simulink model "zrf_test"  (R2019a)
settings: Solver=VariableStepAuto  StartTime=0.0  StopTime=10.0  RelTol=1e-3
libraries: xbsIndex_r4 x3314, casper_library_misc x18, xps_library x3
(part 1 of 32)
settings Model: Creator=jackh  LastModifiedBy=jackh

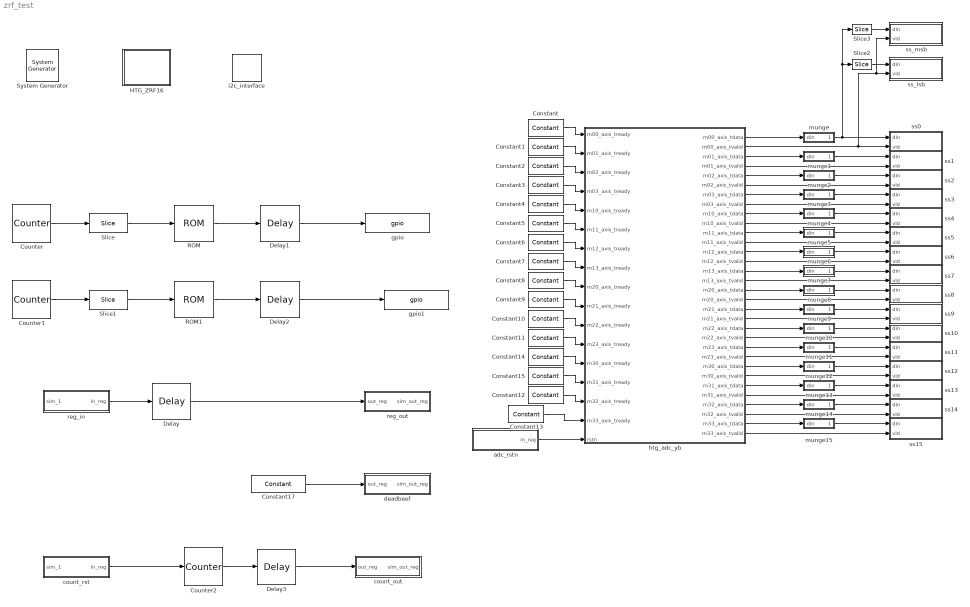
== system zrf_test ==
  " System Generator" : xbsIndex_r4/ System Generator  Tag=genX  xilinxfamily=zynquplusRFSOC  part=xczu49dr  speed=-2-e  package=ffvf1760  synthesis_tool=XST  clock_wrapper=Clock Enables  directory=/home/jackh/src/ata_rfsoc/zrf_test/sysgen  proj_type=Vivado  Synth_file=Vivado Synthesis Defaults  Impl_file=Vivado Implementation Defaults  testbench=off  simulink_period=1  sysclk_period=3.9062  dcm_input_clock_period=10  incr_netlist=off  trim_vbits=Everywhere in SubSystem  dbl_ovrd=According to Block Masks  core_generation=According to Block Masks  run_coregen=off  deprecated_control=off  eval_field=0  block_type=sysgen
  Constant{,1..15} (16 alike) : xbsIndex_r4/Constant  const=1  gui_display_data_type=Boolean  arith_type=Boolean  n_bits=1  bin_pt=0  preci_type=Single  exp_width=8  frac_width=24  explicit_period=on  period=1  equ=P=C  opselect=C  inp2=PCIN>>17  opr=+  inp1=P  carry=CIN  dbl_ovrd=off  block_type=constant
  Constant17 : xbsIndex_r4/Constant  const=hex2dec('deadbeef')  gui_display_data_type=Fixed-point  arith_type=Unsigned  n_bits=32  bin_pt=0  preci_type=Single  exp_width=8  frac_width=24  explicit_period=on  period=1  equ=P=C  opselect=C  inp2=PCIN>>17  opr=+  inp1=P  carry=CIN  dbl_ovrd=off  block_type=constant
  Counter : xbsIndex_r4/Counter  cnt_type=Free Running  cnt_to=Inf  operation=Up  start_count=0  cnt_by_val=1  arith_type=Unsigned  n_bits=32  bin_pt=0  load_pin=off  rst=off  en=off  explicit_period=on  period=1  use_behavioral_HDL=off  implementation=Fabric  dbl_ovrd=off  block_type=counter
  Counter1 : xbsIndex_r4/Counter  cnt_type=Free Running  cnt_to=Inf  operation=Up  start_count=0  cnt_by_val=1  arith_type=Unsigned  n_bits=32  bin_pt=0  load_pin=off  rst=off  en=off  explicit_period=on  period=1  use_behavioral_HDL=off  implementation=Fabric  dbl_ovrd=off  block_type=counter
  Counter2 : xbsIndex_r4/Counter  cnt_type=Free Running  cnt_to=Inf  operation=Up  start_count=0  cnt_by_val=1  arith_type=Unsigned  n_bits=32  bin_pt=0  load_pin=off  rst=on  en=off  explicit_period=on  period=1  use_behavioral_HDL=off  implementation=DSP48  dbl_ovrd=off  block_type=counter
  Delay{,1..3} (4 alike) : xbsIndex_r4/Delay  rst=off  infoeditControl=Selection of Reset will increase slice count due to use of real FFs and instead of SRLs  en=off  latency=1  reg_retiming=off  dbl_ovrd=off  block_type=delay
  HTG_ZRF16 : Subsystem  Tag=xps:xsg  mask(xsg core config){hw_sys=htg_zrf16:xczu49dr, clk_src=adc_clk, clk_rate=256, sample_period=1, synthesis_tool=XST}
      mask prompts: hw_sys "Hardware Platform"; clk_src "User IP Clock source"; clk_rate "User IP Clock Rate (MHz)"; sample_period "Sample Period"; synthesis_tool "Synthesis Tool:"
      mask help:
      | The XSG Core Config block is used to configure the System Generator design
      | for the casper_xps toolflow. Settings here are used to configure the
      | Xilinx System Generator block parameters automatically, and control toolflow
      | script  execution. It needs to be at the top level of all designs being compiled
      | with the casper_xps toolflow.
      mask init:
      | xps_xsg_htg_zrf16_conf_mask;
      mask Help: eval('xlWeb([getenv(''MLIB_ROOT''), ''\doc\html\sys_xsg_core_config\sys_xsg_core_config.html''])')
      mask TypeOptions hw_sys: htg_zrf16:xczu29dr | htg_zrf16:xczu49dr
      mask TypeOptions clk_src: sys_clk | adc_clk | arb_clk
      mask TypeOptions synthesis_tool: Leonardo Spectrum | Synplify | Synplify Pro | XST
      mask Display: fprintf(['ZRF16']);
  ROM : xbsIndex_r4/ROM  depth=16  initVector=[0 1 2 4 8 16 32 64 64 32 16 8 4 2 1 0]  distributed_mem=Distributed memory  rst=off  init_reg=0  en=off  latency=1  gui_display_data_type=Fixed-point  arith_type=Unsigned  n_bits=7  bin_pt=0  preci_type=Single  exp_width=8  frac_width=24  optimize=Area  use_rpm=on  dbl_ovrd=off  simulation_type=fast_sim  block_type=sprom
  ROM1 : xbsIndex_r4/ROM  depth=16  initVector=[1 2 4 8 16 32 64 128 128 64 32 16 8 4 2 1]  distributed_mem=Distributed memory  rst=off  init_reg=0  en=off  latency=1  gui_display_data_type=Fixed-point  arith_type=Unsigned  n_bits=8  bin_pt=0  preci_type=Single  exp_width=8  frac_width=24  optimize=Area  use_rpm=on  dbl_ovrd=off  simulation_type=fast_sim  block_type=sprom
  Slice : xbsIndex_r4/Slice  nbits=4  boolean_output=off  mode=Lower Bit Location + Width  bit1=0  base1=MSB of Input  bit0=25  base0=LSB of Input  dbl_ovrd=off  block_type=slice
  Slice1 : xbsIndex_r4/Slice  nbits=4  boolean_output=off  mode=Lower Bit Location + Width  bit1=0  base1=MSB of Input  bit0=25  base0=LSB of Input  dbl_ovrd=off  block_type=slice
  Slice2 : xbsIndex_r4/Slice  nbits=8  boolean_output=off  mode=Lower Bit Location + Width  bit1=0  base1=MSB of Input  bit0=0  base0=LSB of Input  dbl_ovrd=off  block_type=slice
  Slice3 : xbsIndex_r4/Slice  nbits=8  boolean_output=off  mode=Lower Bit Location + Width  bit1=0  base1=MSB of Input  bit0=8  base0=LSB of Input  dbl_ovrd=off  block_type=slice
  adc_rstn : Subsystem  Tag=xps:sw_reg  AncestorBlock=xps_library/Memory/software_register  mask(swreg){io_dir=From Processor, io_delay=0, init_val=0, sample_period=1, names=reg, bitwidths=1, bin_pts=0, arith_types=2, sim_port=off, show_format=on}
      mask prompts: io_dir "I/O direction"; io_delay "I/O delay"; init_val "Initial Value"; sample_period "Sample period"; names "Bitfield names [msb...lsb]"; bitwidths "Bitfield widths"; bin_pts "Bitfield binary pts"; arith_types "Bitfield types, ufix=0, fix=1, bool=2"; sim_port "Provide sim input/output?"; show_format "Print format string?"
      mask help: A 32-bit software-accessible register. Can be divided into bitfields of varying widths and types using the fields in the block mask.
      mask init:
      | swreg_init(gcb)
      settings: AttributesFormatString=1input:b = 1 bits
      mask TypeOptions io_dir: To Processor | From Processor
      mask Callback io_dir:
      | mask_enables = get_param(gcb, 'MaskEnables');
      | mask_names = get_param(gcb, 'MaskNames');
      | if strcmp(get_param(gcb, 'io_dir'), 'To Processor'),
      |     mask_enables{ismember(mask_names, 'sample_period')} = 'off';
      | else
      |     mask_enables{ismember(mask_names, 'sample_period')} = 'on';
      | end
      | set_param(gcb, 'MaskEnables', mask_enables);
      mask DialogControl ParameterTabVar0 Prompt: Setup
  count_out : Subsystem  Tag=xps:sw_reg  AncestorBlock=xps_library/Memory/software_register  mask(swreg){io_dir=To Processor, io_delay=0, init_val=0, sample_period=1, names=reg, bitwidths=32, bin_pts=0, arith_types=0, sim_port=on, show_format=on}
      mask prompts: io_dir "I/O direction"; io_delay "I/O delay"; init_val "Initial Value"; sample_period "Sample period"; names "Bitfield names [msb...lsb]"; bitwidths "Bitfield widths"; bin_pts "Bitfield binary pts"; arith_types "Bitfield types, ufix=0, fix=1, bool=2"; sim_port "Provide sim input/output?"; show_format "Print format string?"
      mask help: A 32-bit software-accessible register. Can be divided into bitfields of varying widths and types using the fields in the block mask.
      mask init:
      | swreg_init(gcb)
      settings: AttributesFormatString=1output:uf32.0 = 32 bits
      mask TypeOptions io_dir: To Processor | From Processor
      mask Callback io_dir:
      | mask_enables = get_param(gcb, 'MaskEnables');
      | mask_names = get_param(gcb, 'MaskNames');
      | if strcmp(get_param(gcb, 'io_dir'), 'To Processor'),
      |     mask_enables{ismember(mask_names, 'sample_period')} = 'off';
      | else
      |     mask_enables{ismember(mask_names, 'sample_period')} = 'on';
      | end
      | set_param(gcb, 'MaskEnables', mask_enables);
      mask DialogControl ParameterTabVar0 Prompt: Setup
  count_rst : Subsystem  Tag=xps:sw_reg  AncestorBlock=xps_library/Memory/software_register  mask(swreg){io_dir=From Processor, io_delay=0, init_val=0, sample_period=1, names=reg, bitwidths=1, bin_pts=0, arith_types=2, sim_port=on, show_format=on}
      mask prompts: io_dir "I/O direction"; io_delay "I/O delay"; init_val "Initial Value"; sample_period "Sample period"; names "Bitfield names [msb...lsb]"; bitwidths "Bitfield widths"; bin_pts "Bitfield binary pts"; arith_types "Bitfield types, ufix=0, fix=1, bool=2"; sim_port "Provide sim input/output?"; show_format "Print format string?"
      mask help: A 32-bit software-accessible register. Can be divided into bitfields of varying widths and types using the fields in the block mask.
      mask init:
      | swreg_init(gcb)
      settings: AttributesFormatString=1input:b = 1 bits
      mask TypeOptions io_dir: To Processor | From Processor
      mask Callback io_dir:
      | mask_enables = get_param(gcb, 'MaskEnables');
      | mask_names = get_param(gcb, 'MaskNames');
      | if strcmp(get_param(gcb, 'io_dir'), 'To Processor'),
      |     mask_enables{ismember(mask_names, 'sample_period')} = 'off';
      | else
      |     mask_enables{ismember(mask_names, 'sample_period')} = 'on';
      | end
      | set_param(gcb, 'MaskEnables', mask_enables);
      mask DialogControl ParameterTabVar0 Prompt: Setup
  deadbeef : Subsystem  Tag=xps:sw_reg  AncestorBlock=xps_library/Memory/software_register  mask(swreg){io_dir=To Processor, io_delay=0, init_val=0, sample_period=1, names=reg, bitwidths=32, bin_pts=0, arith_types=0, sim_port=on, show_format=on}
      mask prompts: io_dir "I/O direction"; io_delay "I/O delay"; init_val "Initial Value"; sample_period "Sample period"; names "Bitfield names [msb...lsb]"; bitwidths "Bitfield widths"; bin_pts "Bitfield binary pts"; arith_types "Bitfield types, ufix=0, fix=1, bool=2"; sim_port "Provide sim input/output?"; show_format "Print format string?"
      mask help: A 32-bit software-accessible register. Can be divided into bitfields of varying widths and types using the fields in the block mask.
      mask init:
      | swreg_init(gcb)
      settings: AttributesFormatString=1output:uf32.0 = 32 bits
      mask TypeOptions io_dir: To Processor | From Processor
      mask Callback io_dir:
      | mask_enables = get_param(gcb, 'MaskEnables');
      | mask_names = get_param(gcb, 'MaskNames');
      | if strcmp(get_param(gcb, 'io_dir'), 'To Processor'),
      |     mask_enables{ismember(mask_names, 'sample_period')} = 'off';
      | else
      |     mask_enables{ismember(mask_names, 'sample_period')} = 'on';
      | end
      | set_param(gcb, 'MaskEnables', mask_enables);
      mask DialogControl ParameterTabVar0 Prompt: Setup
  gpio : xps_library/IO/gpio  Tag=xps:gpio  io_group_params_forwarded=off  io_group=ROACH:led  io_group_real=led  io_group_custom=0  io_dir=out  arith_type=Unsigned  bitwidth=7  bin_pt=0  bit_index=[0 1 2 3 4 5 6]  sample_period=1  use_single_ended=off  use_ddr=off  reg_iob=on  reg_clk_phase=0  termination=None
      settings: SourceProductName=CASPER XPS Blockset
  gpio1 : xps_library/IO/gpio  Tag=xps:gpio  io_group_params_forwarded=off  io_group=ROACH:led  io_group_real=gpio  io_group_custom=0  io_dir=out  arith_type=Unsigned  bitwidth=8  bin_pt=0  bit_index=[0 1 2 3 4 5 6 7]  sample_period=1  use_single_ended=off  use_ddr=off  reg_iob=on  reg_clk_phase=0  termination=None
      settings: SourceProductName=CASPER XPS Blockset
  htg_adc_yb : Subsystem  Tag=xps:adc_htgzrf16  mask(htg_adc){tile_224_enable_pll=on, tile_224_sample_rate=4096, tile_224_clk_out=256.000, tile_224_ref_clk=512.000, tile_224_axi_stream_clk=0, tile_224_adc_0=on, tile_224_adc0_digital_output=I/Q, tile_224_adc0_dec_mode=2x, tile_224_adc0_sample_per_cycle=8, tile_224_adc0_req_axis_clk=0, tile_224_adc_1=on, tile_224_adc1_digital_output=I/Q, tile_224_adc1_dec_mode=2x, tile_224_adc1_sample_per_cycle=8, tile_224_adc1_req_axis_clk=0, tile_225_enable_pll=on, tile_225_sample_rate=4096, tile_225_clk_out=256.000, tile_225_ref_clk=512.000, tile_225_axi_stream_clk=0, tile_225_adc_0=on, tile_225_adc0_digital_output=I/Q, tile_225_adc0_dec_mode=2x, tile_225_adc0_sample_per_cycle=8, tile_225_adc0_req_axis_clk=0, tile_225_adc_1=on, tile_225_adc1_digital_output=I/Q, tile_225_adc1_dec_mode=2x, tile_225_adc1_sample_per_cycle=8, tile_225_adc1_req_axis_clk=0, tile_226_enable_pll=on, tile_226_sample_rate=4096, tile_226_clk_out=256.000, tile_226_ref_clk=512.000, tile_226_axi_stream_clk=0, tile_226_adc_0=on, tile_226_adc0_digital_output=I/Q, tile_226_adc0_dec_mode=2x, tile_226_adc0_sample_per_cycle=8, tile_226_adc0_req_axis_clk=0, tile_226_adc_1=on, tile_226_adc1_digital_output=I/Q, tile_226_adc1_dec_mode=2x, tile_226_adc1_sample_per_cycle=8, tile_226_adc1_req_axis_clk=0, tile_227_enable_pll=on, tile_227_sample_rate=4096, tile_227_clk_out=256.000, tile_227_ref_clk=512.000, tile_227_axi_stream_clk=0, tile_227_adc_0=on, tile_227_adc0_digital_output=I/Q, tile_227_adc0_dec_mode=2x, tile_227_adc0_sample_per_cycle=8, tile_227_adc0_req_axis_clk=0, tile_227_adc_1=on, tile_227_adc1_digital_output=I/Q, tile_227_adc1_dec_mode=2x, tile_227_adc1_sample_per_cycle=8, tile_227_adc1_req_axis_clk=0}
      mask prompts: tile_224_enable_pll "Enable PLL"; tile_224_sample_rate "Sampling Rate (MSPS)"; tile_224_clk_out "Clock Out (MHz)"; tile_224_ref_clk "Reference Clock (MHz)"; tile_224_axi_stream_clk "AXI4-Stream Clock (MHz)"; tile_224_adc_0 "Enable ADC"; tile_224_adc0_digital_output "Digital Output Data"; tile_224_adc0_dec_mode "Decimation Mode"; tile_224_adc0_sample_per_cycle "Samples per AXI4-Stream Cycle"; tile_224_adc_1 "Enable ADC"; tile_224_adc1_digital_output "Digital Output Data"; tile_224_adc1_dec_mode "Decimation Mode"; tile_224_adc1_sample_per_cycle "Samples per AXI4-Stream Cycle"; tile_225_enable_pll "Enable PLL"; tile_225_sample_rate "Sampling Rate (MSPS)"; tile_225_clk_out "Clock Out (MHz)"; tile_225_ref_clk "Reference Clock (MHz)"; tile_225_axi_stream_clk "AXI4-Stream Clock (MHz)"; tile_225_adc_0 "Enable ADC"; tile_225_adc0_digital_output "Digital Output Data"; tile_225_adc0_dec_mode "Decimation Mode"; tile_225_adc0_sample_per_cycle "Samples per AXI4-Stream Cycle"; tile_225_adc_1 "Enable ADC"; tile_225_adc1_digital_output "Digital Output Data"; tile_225_adc1_dec_mode "Decimation Mode"; tile_225_adc1_sample_per_cycle "Samples per AXI4-Stream Cycle"; tile_226_enable_pll "Enable PLL"; tile_226_sample_rate "Sampling Rate (MSPS)"; tile_226_clk_out "Clock Out (MHz)"; tile_226_ref_clk "Reference Clock (MHz)"; tile_226_axi_stream_clk "AXI4-Stream Clock (MHz)"; tile_226_adc_0 "Enable ADC"; tile_226_adc0_digital_output "Digital Output Data"; tile_226_adc0_dec_mode "Decimation Mode"; tile_226_adc0_sample_per_cycle "Samples per AXI4-Stream Cycle"; tile_226_adc_1 "Enable ADC"; tile_226_adc1_digital_output "Digital Output Data"; tile_226_adc1_dec_mode "Decimation Mode"; tile_226_adc1_sample_per_cycle "Samples per AXI4-Stream Cycle"; tile_227_enable_pll "Enable PLL"; tile_227_sample_rate "Sampling Rate (MSPS)"; tile_227_clk_out "Clock Out (MHz)"; tile_227_ref_clk "Reference Clock (MHz)"; tile_227_axi_stream_clk "AXI4-Stream Clock (MHz)"; tile_227_adc_0 "Enable ADC"; tile_227_adc0_digital_output "Digital Output Data"; tile_227_adc0_dec_mode "Decimation Mode"; tile_227_adc0_sample_per_cycle "Samples per AXI4-Stream Cycle"; tile_227_adc_1 "Enable ADC"; tile_227_adc1_digital_output "Digital Output Data"; tile_227_adc1_dec_mode "Decimation Mode"; tile_227_adc1_sample_per_cycle "Samples per AXI4-Stream Cycle"
      mask init:
      | htg_adc_mask(gcb)
      mask Help: eval('xlWeb([getenv(''MLIB_ROOT''), ''\doc\html\adc_zcu111\adc_zcu111.html''])')
      mask TypeOptions tile_224_clk_out: 32.000 | 64.000 | 128.000 | 256.000
      mask TypeOptions tile_224_ref_clk: 103.261 | 104.136 | 105.026 | 105.931 | 106.852 | 107.790 | 108.743 | 109.714 | 110.703 | 111.709 | 112.734 | 113.778 | 114.841 | 115.925 | 117.029 | 118.154 | 119.301 | 120.471 | 121.663 | 122.880 | 124.121 | 125.388 | 126.680 | 128.000 | 129.347 | 130.723 | 132.129 | 133.565 | 135.033 | 136.533 | 138.067 | 139.636 | 141.241 | 142.884 | 144.565 | 146.286 | 148.048 | 149.854 | 151.704 | 153.600 | 155.544 | 157.539 | 159.584 | 161.684 | 163.840 | 166.054 | 168.329 | 170.667 | 173.070 | 175.543 | 178.087 | 180.706 | 183.403 | 186.182 | 189.046 | 192.000 | 195.048 | 198.194 | 201.443 | 204.800 | 208.271 | 211.862 | 215.579 | 219.429 | 223.418 | 227.556 | 231.849 | 236.308 | 240.941 | 245.760 | 250.776 | 256.000 | 261.447 | 267.130 | 273.067 | 279.273 | 285.767 | 292.571 | 299.707 | 307.200 | 315.077 | 323.368 | 332.108 | 341.333 | 351.086 | 361.412 | 372.364 | 384.000 | 396.387 | 409.600 | 423.724 | 438.857 | 455.111 | 472.615 | 491.520 | 512.000 | 534.261 | 558.546 | 585.143 | 614.400 | 646.737 | 682.667 | 722.824 | 768.000
      mask TypeOptions tile_224_adc0_digital_output: I/Q | Real
      mask TypeOptions tile_224_adc0_dec_mode: 1x | 2x | 4x | 8x
      mask TypeOptions tile_224_adc0_sample_per_cycle: 1 | 2 | 3 | 4 | 5 | 6 | 7 | 8
      mask TypeOptions tile_224_adc1_digital_output: I/Q | Real
      mask TypeOptions tile_224_adc1_dec_mode: 1x | 2x | 4x | 8x
      mask TypeOptions tile_224_adc1_sample_per_cycle: 1 | 2 | 3 | 4 | 5 | 6 | 7 | 8
      mask TypeOptions tile_225_clk_out: 32.000 | 64.000 | 128.000 | 256.000
      mask TypeOptions tile_225_ref_clk: 103.261 | 104.136 | 105.026 | 105.931 | 106.852 | 107.790 | 108.743 | 109.714 | 110.703 | 111.709 | 112.734 | 113.778 | 114.841 | 115.925 | 117.029 | 118.154 | 119.301 | 120.471 | 121.663 | 122.880 | 124.121 | 125.388 | 126.680 | 128.000 | 129.347 | 130.723 | 132.129 | 133.565 | 135.033 | 136.533 | 138.067 | 139.636 | 141.241 | 142.884 | 144.565 | 146.286 | 148.048 | 149.854 | 151.704 | 153.600 | 155.544 | 157.539 | 159.584 | 161.684 | 163.840 | 166.054 | 168.329 | 170.667 | 173.070 | 175.543 | 178.087 | 180.706 | 183.403 | 186.182 | 189.046 | 192.000 | 195.048 | 198.194 | 201.443 | 204.800 | 208.271 | 211.862 | 215.579 | 219.429 | 223.418 | 227.556 | 231.849 | 236.308 | 240.941 | 245.760 | 250.776 | 256.000 | 261.447 | 267.130 | 273.067 | 279.273 | 285.767 | 292.571 | 299.707 | 307.200 | 315.077 | 323.368 | 332.108 | 341.333 | 351.086 | 361.412 | 372.364 | 384.000 | 396.387 | 409.600 | 423.724 | 438.857 | 455.111 | 472.615 | 491.520 | 512.000 | 534.261 | 558.546 | 585.143 | 614.400 | 646.737 | 682.667 | 722.824 | 768.000
      mask TypeOptions tile_225_adc0_digital_output: I/Q | Real
      mask TypeOptions tile_225_adc0_dec_mode: 1x | 2x | 4x | 8x
      mask TypeOptions tile_225_adc0_sample_per_cycle: 1 | 2 | 3 | 4 | 5 | 6 | 7 | 8
      mask TypeOptions tile_225_adc1_digital_output: I/Q | Real
      mask TypeOptions tile_225_adc1_dec_mode: 1x | 2x | 4x | 8x
      mask TypeOptions tile_225_adc1_sample_per_cycle: 1 | 2 | 3 | 4 | 5 | 6 | 7 | 8
      mask TypeOptions tile_226_clk_out: 32.000 | 64.000 | 128.000 | 256.000
      mask TypeOptions tile_226_ref_clk: 103.261 | 104.136 | 105.026 | 105.931 | 106.852 | 107.790 | 108.743 | 109.714 | 110.703 | 111.709 | 112.734 | 113.778 | 114.841 | 115.925 | 117.029 | 118.154 | 119.301 | 120.471 | 121.663 | 122.880 | 124.121 | 125.388 | 126.680 | 128.000 | 129.347 | 130.723 | 132.129 | 133.565 | 135.033 | 136.533 | 138.067 | 139.636 | 141.241 | 142.884 | 144.565 | 146.286 | 148.048 | 149.854 | 151.704 | 153.600 | 155.544 | 157.539 | 159.584 | 161.684 | 163.840 | 166.054 | 168.329 | 170.667 | 173.070 | 175.543 | 178.087 | 180.706 | 183.403 | 186.182 | 189.046 | 192.000 | 195.048 | 198.194 | 201.443 | 204.800 | 208.271 | 211.862 | 215.579 | 219.429 | 223.418 | 227.556 | 231.849 | 236.308 | 240.941 | 245.760 | 250.776 | 256.000 | 261.447 | 267.130 | 273.067 | 279.273 | 285.767 | 292.571 | 299.707 | 307.200 | 315.077 | 323.368 | 332.108 | 341.333 | 351.086 | 361.412 | 372.364 | 384.000 | 396.387 | 409.600 | 423.724 | 438.857 | 455.111 | 472.615 | 491.520 | 512.000 | 534.261 | 558.546 | 585.143 | 614.400 | 646.737 | 682.667 | 722.824 | 768.000
      mask TypeOptions tile_226_adc0_digital_output: I/Q | Real
      mask TypeOptions tile_226_adc0_dec_mode: 1x | 2x | 4x | 8x
      mask TypeOptions tile_226_adc0_sample_per_cycle: 1 | 2 | 3 | 4 | 5 | 6 | 7 | 8
      mask TypeOptions tile_226_adc1_digital_output: I/Q | Real
      mask TypeOptions tile_226_adc1_dec_mode: 1x | 2x | 4x | 8x
      mask TypeOptions tile_226_adc1_sample_per_cycle: 1 | 2 | 3 | 4 | 5 | 6 | 7 | 8
      mask TypeOptions tile_227_clk_out: 32.000 | 64.000 | 128.000 | 256.000
      mask TypeOptions tile_227_ref_clk: 103.261 | 104.136 | 105.026 | 105.931 | 106.852 | 107.790 | 108.743 | 109.714 | 110.703 | 111.709 | 112.734 | 113.778 | 114.841 | 115.925 | 117.029 | 118.154 | 119.301 | 120.471 | 121.663 | 122.880 | 124.121 | 125.388 | 126.680 | 128.000 | 129.347 | 130.723 | 132.129 | 133.565 | 135.033 | 136.533 | 138.067 | 139.636 | 141.241 | 142.884 | 144.565 | 146.286 | 148.048 | 149.854 | 151.704 | 153.600 | 155.544 | 157.539 | 159.584 | 161.684 | 163.840 | 166.054 | 168.329 | 170.667 | 173.070 | 175.543 | 178.087 | 180.706 | 183.403 | 186.182 | 189.046 | 192.000 | 195.048 | 198.194 | 201.443 | 204.800 | 208.271 | 211.862 | 215.579 | 219.429 | 223.418 | 227.556 | 231.849 | 236.308 | 240.941 | 245.760 | 250.776 | 256.000 | 261.447 | 267.130 | 273.067 | 279.273 | 285.767 | 292.571 | 299.707 | 307.200 | 315.077 | 323.368 | 332.108 | 341.333 | 351.086 | 361.412 | 372.364 | 384.000 | 396.387 | 409.600 | 423.724 | 438.857 | 455.111 | 472.615 | 491.520 | 512.000 | 534.261 | 558.546 | 585.143 | 614.400 | 646.737 | 682.667 | 722.824 | 768.000
      mask TypeOptions tile_227_adc0_digital_output: I/Q | Real
      mask TypeOptions tile_227_adc0_dec_mode: 1x | 2x | 4x | 8x
      mask TypeOptions tile_227_adc0_sample_per_cycle: 1 | 2 | 3 | 4 | 5 | 6 | 7 | 8
      mask TypeOptions tile_227_adc1_digital_output: I/Q | Real
      mask TypeOptions tile_227_adc1_dec_mode: 1x | 2x | 4x | 8x
      mask TypeOptions tile_227_adc1_sample_per_cycle: 1 | 2 | 3 | 4 | 5 | 6 | 7 | 8
      mask DialogControl adc_tile_224 Prompt: ADC Tile 224
      mask DialogControl pll_clocking_config_224 Prompt: PLL and Clocking Configuration
      mask DialogControl tile_224_adc0 Prompt: ADC 0
      mask DialogControl tile_224_adc0_data_settings Prompt: Data Settings
      mask DialogControl tile_224_adc0_req_axis_clk_label Prompt: Required AXI4-Stream clock:
      mask DialogControl tile_224_adc1 Prompt: ADC 1
      mask DialogControl tile_224_adc1_data_settings Prompt: Data Settings
      mask DialogControl tile_224_adc1_req_axis_clk_label Prompt: Required AXI4-Stream clock:
      mask DialogControl adc_tile_225 Prompt: ADC Tile 225
      mask DialogControl pll_clocking_config_225 Prompt: PLL and Clocking Configuration
      mask DialogControl tile_225_adc0 Prompt: ADC 0
      mask DialogControl tile_225_adc0_data_settings Prompt: Data Settings
      mask DialogControl tile_225_adc0_req_axis_clk_label Prompt: Required AXI4-Stream clock:
      mask DialogControl tile_225_adc1 Prompt: ADC 1
      mask DialogControl tile_225_adc1_data_settings Prompt: Data Settings
      mask DialogControl tile_225_adc1_req_axis_clk_label Prompt: Required AXI4-Stream clock:
      mask DialogControl adc_tile_226 Prompt: ADC Tile 226
      mask DialogControl pll_clocking_config_226 Prompt: PLL and Clocking Configuration
      mask DialogControl tile_226_adc0 Prompt: ADC 0
      mask DialogControl tile_226_adc0_data_settings Prompt: Data Settings
      mask DialogControl tile_226_adc0_req_axis_clk_label Prompt: Required AXI4-Stream clock:
      mask DialogControl tile_226_adc1 Prompt: ADC 1
      mask DialogControl tile_226_adc1_data_settings Prompt: Data Settings
      mask DialogControl tile_226_adc1_req_axis_clk_label Prompt: Required AXI4-Stream clock:
      mask DialogControl adc_tile_227 Prompt: ADC Tile 227
      mask DialogControl pll_clocking_config_227 Prompt: PLL and Clocking Configuration
      mask DialogControl tile_227_adc0 Prompt: ADC 0
      mask DialogControl tile_227_adc0_data_settings Prompt: Data Settings
      mask DialogControl tile_227_adc0_req_axis_clk_label Prompt: Required AXI4-Stream clock:
      mask DialogControl tile_227_adc1 Prompt: ADC 1
      mask DialogControl tile_227_adc1_data_settings Prompt: Data Settings
      mask DialogControl tile_227_adc1_req_axis_clk_label Prompt: Required AXI4-Stream clock:
  i2c_interface : xps_library/IO/i2c_interface  Tag=xps:i2c_interface  sda_gpio='i2c'  sda_gpio_index=0  scl_gpio='i2c'  scl_gpio_index=1
      settings: SourceProductName=CASPER XPS Blockset
  munge : Subsystem  AncestorBlock=casper_library_flow_control/munge  mask(munge){divisions=8, div_size=[16 16 16 16 16 16 16 16], order=[7 6 5 4 3 2 1 0], arith_type_out=Unsigned, bin_pt_out=0}
      mask prompts: divisions "Number of divisions"; div_size "Division size (bits)"; order "Division packing order"; arith_type_out "Output arithmetic type"; bin_pt_out "Output binary point"
      mask help: Splits an input bus into the specified number of divisions and then recombines them in the order specified (most significant division = 0,least = number divisions-1)
      mask init:
      | munge_init(gcb, ...
      |     'divisions', divisions, ...
      |     'div_size', div_size, ...
      |     'order', order, ...
      |     'arith_type_out', arith_type_out, ...
      |     'bin_pt_out', bin_pt_out);
      settings: AttributesFormatString=|
      | split:[16 16 16 16 16 16 16 16]
      | join:[7 6 5 4 3 2 1 0]
      | Unsigned [128,0]
      mask TypeOptions arith_type_out: Unsigned | Signed  (2's comp) | Floating-point
  munge1 : Subsystem  AncestorBlock=casper_library_flow_control/munge  mask(munge){divisions=8, div_size=[16 16 16 16 16 16 16 16], order=[7 6 5 4 3 2 1 0], arith_type_out=Unsigned, bin_pt_out=0}
      mask prompts: divisions "Number of divisions"; div_size "Division size (bits)"; order "Division packing order"; arith_type_out "Output arithmetic type"; bin_pt_out "Output binary point"
      mask help: Splits an input bus into the specified number of divisions and then recombines them in the order specified (most significant division = 0,least = number divisions-1)
      mask init:
      | munge_init(gcb, ...
      |     'divisions', divisions, ...
      |     'div_size', div_size, ...
      |     'order', order, ...
      |     'arith_type_out', arith_type_out, ...
      |     'bin_pt_out', bin_pt_out);
      settings: AttributesFormatString=|
      | split:[16 16 16 16 16 16 16 16]
      | join:[7 6 5 4 3 2 1 0]
      | Unsigned [128,0]
      mask TypeOptions arith_type_out: Unsigned | Signed  (2's comp) | Floating-point
  munge10 : Subsystem  AncestorBlock=casper_library_flow_control/munge  mask(munge){divisions=8, div_size=[16 16 16 16 16 16 16 16], order=[7 6 5 4 3 2 1 0], arith_type_out=Unsigned, bin_pt_out=0}
      mask prompts: divisions "Number of divisions"; div_size "Division size (bits)"; order "Division packing order"; arith_type_out "Output arithmetic type"; bin_pt_out "Output binary point"
      mask help: Splits an input bus into the specified number of divisions and then recombines them in the order specified (most significant division = 0,least = number divisions-1)
      mask init:
      | munge_init(gcb, ...
      |     'divisions', divisions, ...
      |     'div_size', div_size, ...
      |     'order', order, ...
      |     'arith_type_out', arith_type_out, ...
      |     'bin_pt_out', bin_pt_out);
      settings: AttributesFormatString=|
      | split:[16 16 16 16 16 16 16 16]
      | join:[7 6 5 4 3 2 1 0]
      | Unsigned [128,0]
      mask TypeOptions arith_type_out: Unsigned | Signed  (2's comp) | Floating-point
  munge11 : Subsystem  AncestorBlock=casper_library_flow_control/munge  mask(munge){divisions=8, div_size=[16 16 16 16 16 16 16 16], order=[7 6 5 4 3 2 1 0], arith_type_out=Unsigned, bin_pt_out=0}
      mask prompts: divisions "Number of divisions"; div_size "Division size (bits)"; order "Division packing order"; arith_type_out "Output arithmetic type"; bin_pt_out "Output binary point"
      mask help: Splits an input bus into the specified number of divisions and then recombines them in the order specified (most significant division = 0,least = number divisions-1)
      mask init:
      | munge_init(gcb, ...
      |     'divisions', divisions, ...
      |     'div_size', div_size, ...
      |     'order', order, ...
      |     'arith_type_out', arith_type_out, ...
      |     'bin_pt_out', bin_pt_out);
      settings: AttributesFormatString=|
      | split:[16 16 16 16 16 16 16 16]
      | join:[7 6 5 4 3 2 1 0]
      | Unsigned [128,0]
      mask TypeOptions arith_type_out: Unsigned | Signed  (2's comp) | Floating-point
  munge12 : Subsystem  AncestorBlock=casper_library_flow_control/munge  mask(munge){divisions=8, div_size=[16 16 16 16 16 16 16 16], order=[7 6 5 4 3 2 1 0], arith_type_out=Unsigned, bin_pt_out=0}
      mask prompts: divisions "Number of divisions"; div_size "Division size (bits)"; order "Division packing order"; arith_type_out "Output arithmetic type"; bin_pt_out "Output binary point"
      mask help: Splits an input bus into the specified number of divisions and then recombines them in the order specified (most significant division = 0,least = number divisions-1)
      mask init:
      | munge_init(gcb, ...
      |     'divisions', divisions, ...
      |     'div_size', div_size, ...
      |     'order', order, ...
      |     'arith_type_out', arith_type_out, ...
      |     'bin_pt_out', bin_pt_out);
      settings: AttributesFormatString=|
      | split:[16 16 16 16 16 16 16 16]
      | join:[7 6 5 4 3 2 1 0]
      | Unsigned [128,0]
      mask TypeOptions arith_type_out: Unsigned | Signed  (2's comp) | Floating-point
  munge13 : Subsystem  AncestorBlock=casper_library_flow_control/munge  mask(munge){divisions=8, div_size=[16 16 16 16 16 16 16 16], order=[7 6 5 4 3 2 1 0], arith_type_out=Unsigned, bin_pt_out=0}
      mask prompts: divisions "Number of divisions"; div_size "Division size (bits)"; order "Division packing order"; arith_type_out "Output arithmetic type"; bin_pt_out "Output binary point"
      mask help: Splits an input bus into the specified number of divisions and then recombines them in the order specified (most significant division = 0,least = number divisions-1)
      mask init:
      | munge_init(gcb, ...
      |     'divisions', divisions, ...
      |     'div_size', div_size, ...
      |     'order', order, ...
      |     'arith_type_out', arith_type_out, ...
      |     'bin_pt_out', bin_pt_out);
      settings: AttributesFormatString=|
      | split:[16 16 16 16 16 16 16 16]
      | join:[7 6 5 4 3 2 1 0]
      | Unsigned [128,0]
      mask TypeOptions arith_type_out: Unsigned | Signed  (2's comp) | Floating-point
  munge14 : Subsystem  AncestorBlock=casper_library_flow_control/munge  mask(munge){divisions=8, div_size=[16 16 16 16 16 16 16 16], order=[7 6 5 4 3 2 1 0], arith_type_out=Unsigned, bin_pt_out=0}
      mask prompts: divisions "Number of divisions"; div_size "Division size (bits)"; order "Division packing order"; arith_type_out "Output arithmetic type"; bin_pt_out "Output binary point"
      mask help: Splits an input bus into the specified number of divisions and then recombines them in the order specified (most significant division = 0,least = number divisions-1)
      mask init:
      | munge_init(gcb, ...
      |     'divisions', divisions, ...
      |     'div_size', div_size, ...
      |     'order', order, ...
      |     'arith_type_out', arith_type_out, ...
      |     'bin_pt_out', bin_pt_out);
      settings: AttributesFormatString=|
      | split:[16 16 16 16 16 16 16 16]
      | join:[7 6 5 4 3 2 1 0]
      | Unsigned [128,0]
      mask TypeOptions arith_type_out: Unsigned | Signed  (2's comp) | Floating-point
  munge15 : Subsystem  AncestorBlock=casper_library_flow_control/munge  mask(munge){divisions=8, div_size=[16 16 16 16 16 16 16 16], order=[7 6 5 4 3 2 1 0], arith_type_out=Unsigned, bin_pt_out=0}
      mask prompts: divisions "Number of divisions"; div_size "Division size (bits)"; order "Division packing order"; arith_type_out "Output arithmetic type"; bin_pt_out "Output binary point"
      mask help: Splits an input bus into the specified number of divisions and then recombines them in the order specified (most significant division = 0,least = number divisions-1)
      mask init:
      | munge_init(gcb, ...
      |     'divisions', divisions, ...
      |     'div_size', div_size, ...
      |     'order', order, ...
      |     'arith_type_out', arith_type_out, ...
      |     'bin_pt_out', bin_pt_out);
      settings: AttributesFormatString=|
      | split:[16 16 16 16 16 16 16 16]
      | join:[7 6 5 4 3 2 1 0]
      | Unsigned [128,0]
      mask TypeOptions arith_type_out: Unsigned | Signed  (2's comp) | Floating-point
  munge2 : Subsystem  AncestorBlock=casper_library_flow_control/munge  mask(munge){divisions=8, div_size=[16 16 16 16 16 16 16 16], order=[7 6 5 4 3 2 1 0], arith_type_out=Unsigned, bin_pt_out=0}
      mask prompts: divisions "Number of divisions"; div_size "Division size (bits)"; order "Division packing order"; arith_type_out "Output arithmetic type"; bin_pt_out "Output binary point"
      mask help: Splits an input bus into the specified number of divisions and then recombines them in the order specified (most significant division = 0,least = number divisions-1)
      mask init:
      | munge_init(gcb, ...
      |     'divisions', divisions, ...
      |     'div_size', div_size, ...
      |     'order', order, ...
      |     'arith_type_out', arith_type_out, ...
      |     'bin_pt_out', bin_pt_out);
      settings: AttributesFormatString=|
      | split:[16 16 16 16 16 16 16 16]
      | join:[7 6 5 4 3 2 1 0]
      | Unsigned [128,0]
      mask TypeOptions arith_type_out: Unsigned | Signed  (2's comp) | Floating-point
  munge3 : Subsystem  AncestorBlock=casper_library_flow_control/munge  mask(munge){divisions=8, div_size=[16 16 16 16 16 16 16 16], order=[7 6 5 4 3 2 1 0], arith_type_out=Unsigned, bin_pt_out=0}
      mask prompts: divisions "Number of divisions"; div_size "Division size (bits)"; order "Division packing order"; arith_type_out "Output arithmetic type"; bin_pt_out "Output binary point"
      mask help: Splits an input bus into the specified number of divisions and then recombines them in the order specified (most significant division = 0,least = number divisions-1)
      mask init:
      | munge_init(gcb, ...
      |     'divisions', divisions, ...
      |     'div_size', div_size, ...
      |     'order', order, ...
      |     'arith_type_out', arith_type_out, ...
      |     'bin_pt_out', bin_pt_out);
      settings: AttributesFormatString=|
      | split:[16 16 16 16 16 16 16 16]
      | join:[7 6 5 4 3 2 1 0]
      | Unsigned [128,0]
      mask TypeOptions arith_type_out: Unsigned | Signed  (2's comp) | Floating-point
  munge4 : Subsystem  AncestorBlock=casper_library_flow_control/munge  mask(munge){divisions=8, div_size=[16 16 16 16 16 16 16 16], order=[7 6 5 4 3 2 1 0], arith_type_out=Unsigned, bin_pt_out=0}
      mask prompts: divisions "Number of divisions"; div_size "Division size (bits)"; order "Division packing order"; arith_type_out "Output arithmetic type"; bin_pt_out "Output binary point"
      mask help: Splits an input bus into the specified number of divisions and then recombines them in the order specified (most significant division = 0,least = number divisions-1)
      mask init:
      | munge_init(gcb, ...
      |     'divisions', divisions, ...
      |     'div_size', div_size, ...
      |     'order', order, ...
      |     'arith_type_out', arith_type_out, ...
      |     'bin_pt_out', bin_pt_out);
      settings: AttributesFormatString=|
      | split:[16 16 16 16 16 16 16 16]
      | join:[7 6 5 4 3 2 1 0]
      | Unsigned [128,0]
      mask TypeOptions arith_type_out: Unsigned | Signed  (2's comp) | Floating-point
  munge5 : Subsystem  AncestorBlock=casper_library_flow_control/munge  mask(munge){divisions=8, div_size=[16 16 16 16 16 16 16 16], order=[7 6 5 4 3 2 1 0], arith_type_out=Unsigned, bin_pt_out=0}
      mask prompts: divisions "Number of divisions"; div_size "Division size (bits)"; order "Division packing order"; arith_type_out "Output arithmetic type"; bin_pt_out "Output binary point"
      mask help: Splits an input bus into the specified number of divisions and then recombines them in the order specified (most significant division = 0,least = number divisions-1)
      mask init:
      | munge_init(gcb, ...
      |     'divisions', divisions, ...
      |     'div_size', div_size, ...
      |     'order', order, ...
      |     'arith_type_out', arith_type_out, ...
      |     'bin_pt_out', bin_pt_out);
      settings: AttributesFormatString=|
      | split:[16 16 16 16 16 16 16 16]
      | join:[7 6 5 4 3 2 1 0]
      | Unsigned [128,0]
      mask TypeOptions arith_type_out: Unsigned | Signed  (2's comp) | Floating-point
  munge6 : Subsystem  AncestorBlock=casper_library_flow_control/munge  mask(munge){divisions=8, div_size=[16 16 16 16 16 16 16 16], order=[7 6 5 4 3 2 1 0], arith_type_out=Unsigned, bin_pt_out=0}
      mask prompts: divisions "Number of divisions"; div_size "Division size (bits)"; order "Division packing order"; arith_type_out "Output arithmetic type"; bin_pt_out "Output binary point"
      mask help: Splits an input bus into the specified number of divisions and then recombines them in the order specified (most significant division = 0,least = number divisions-1)
      mask init:
      | munge_init(gcb, ...
      |     'divisions', divisions, ...
      |     'div_size', div_size, ...
      |     'order', order, ...
      |     'arith_type_out', arith_type_out, ...
      |     'bin_pt_out', bin_pt_out);
      settings: AttributesFormatString=|
      | split:[16 16 16 16 16 16 16 16]
      | join:[7 6 5 4 3 2 1 0]
      | Unsigned [128,0]
      mask TypeOptions arith_type_out: Unsigned | Signed  (2's comp) | Floating-point
  munge7 : Subsystem  AncestorBlock=casper_library_flow_control/munge  mask(munge){divisions=8, div_size=[16 16 16 16 16 16 16 16], order=[7 6 5 4 3 2 1 0], arith_type_out=Unsigned, bin_pt_out=0}
      mask prompts: divisions "Number of divisions"; div_size "Division size (bits)"; order "Division packing order"; arith_type_out "Output arithmetic type"; bin_pt_out "Output binary point"
      mask help: Splits an input bus into the specified number of divisions and then recombines them in the order specified (most significant division = 0,least = number divisions-1)
      mask init:
      | munge_init(gcb, ...
      |     'divisions', divisions, ...
      |     'div_size', div_size, ...
      |     'order', order, ...
      |     'arith_type_out', arith_type_out, ...
      |     'bin_pt_out', bin_pt_out);
      settings: AttributesFormatString=|
      | split:[16 16 16 16 16 16 16 16]
      | join:[7 6 5 4 3 2 1 0]
      | Unsigned [128,0]
      mask TypeOptions arith_type_out: Unsigned | Signed  (2's comp) | Floating-point
  munge8 : Subsystem  AncestorBlock=casper_library_flow_control/munge  mask(munge){divisions=8, div_size=[16 16 16 16 16 16 16 16], order=[7 6 5 4 3 2 1 0], arith_type_out=Unsigned, bin_pt_out=0}
      mask prompts: divisions "Number of divisions"; div_size "Division size (bits)"; order "Division packing order"; arith_type_out "Output arithmetic type"; bin_pt_out "Output binary point"
      mask help: Splits an input bus into the specified number of divisions and then recombines them in the order specified (most significant division = 0,least = number divisions-1)
      mask init:
      | munge_init(gcb, ...
      |     'divisions', divisions, ...
      |     'div_size', div_size, ...
      |     'order', order, ...
      |     'arith_type_out', arith_type_out, ...
      |     'bin_pt_out', bin_pt_out);
      settings: AttributesFormatString=|
      | split:[16 16 16 16 16 16 16 16]
      | join:[7 6 5 4 3 2 1 0]
      | Unsigned [128,0]
      mask TypeOptions arith_type_out: Unsigned | Signed  (2's comp) | Floating-point
  munge9 : Subsystem  AncestorBlock=casper_library_flow_control/munge  mask(munge){divisions=8, div_size=[16 16 16 16 16 16 16 16], order=[7 6 5 4 3 2 1 0], arith_type_out=Unsigned, bin_pt_out=0}
      mask prompts: divisions "Number of divisions"; div_size "Division size (bits)"; order "Division packing order"; arith_type_out "Output arithmetic type"; bin_pt_out "Output binary point"
      mask help: Splits an input bus into the specified number of divisions and then recombines them in the order specified (most significant division = 0,least = number divisions-1)
      mask init:
      | munge_init(gcb, ...
      |     'divisions', divisions, ...
      |     'div_size', div_size, ...
      |     'order', order, ...
      |     'arith_type_out', arith_type_out, ...
      |     'bin_pt_out', bin_pt_out);
      settings: AttributesFormatString=|
      | split:[16 16 16 16 16 16 16 16]
      | join:[7 6 5 4 3 2 1 0]
      | Unsigned [128,0]
      mask TypeOptions arith_type_out: Unsigned | Signed  (2's comp) | Floating-point
  reg_in : Subsystem  Tag=xps:sw_reg  AncestorBlock=xps_library/Memory/software_register  mask(swreg){io_dir=From Processor, io_delay=0, init_val=0, sample_period=1, names=reg, bitwidths=32, bin_pts=0, arith_types=0, sim_port=on, show_format=on}
      mask prompts: io_dir "I/O direction"; io_delay "I/O delay"; init_val "Initial Value"; sample_period "Sample period"; names "Bitfield names [msb...lsb]"; bitwidths "Bitfield widths"; bin_pts "Bitfield binary pts"; arith_types "Bitfield types, ufix=0, fix=1, bool=2"; sim_port "Provide sim input/output?"; show_format "Print format string?"
      mask help: A 32-bit software-accessible register. Can be divided into bitfields of varying widths and types using the fields in the block mask.
      mask init:
      | swreg_init(gcb)
      settings: AttributesFormatString=1input:uf32.0 = 32 bits
      mask TypeOptions io_dir: To Processor | From Processor
      mask Callback io_dir:
      | mask_enables = get_param(gcb, 'MaskEnables');
      | mask_names = get_param(gcb, 'MaskNames');
      | if strcmp(get_param(gcb, 'io_dir'), 'To Processor'),
      |     mask_enables{ismember(mask_names, 'sample_period')} = 'off';
      | else
      |     mask_enables{ismember(mask_names, 'sample_period')} = 'on';
      | end
      | set_param(gcb, 'MaskEnables', mask_enables);
      mask DialogControl ParameterTabVar0 Prompt: Setup
  reg_out : Subsystem  Tag=xps:sw_reg  AncestorBlock=xps_library/Memory/software_register  mask(swreg){io_dir=To Processor, io_delay=0, init_val=0, sample_period=1, names=reg, bitwidths=32, bin_pts=0, arith_types=0, sim_port=on, show_format=on}
      mask prompts: io_dir "I/O direction"; io_delay "I/O delay"; init_val "Initial Value"; sample_period "Sample period"; names "Bitfield names [msb...lsb]"; bitwidths "Bitfield widths"; bin_pts "Bitfield binary pts"; arith_types "Bitfield types, ufix=0, fix=1, bool=2"; sim_port "Provide sim input/output?"; show_format "Print format string?"
      mask help: A 32-bit software-accessible register. Can be divided into bitfields of varying widths and types using the fields in the block mask.
      mask init:
      | swreg_init(gcb)
      settings: AttributesFormatString=1output:uf32.0 = 32 bits
      mask TypeOptions io_dir: To Processor | From Processor
      mask Callback io_dir:
      | mask_enables = get_param(gcb, 'MaskEnables');
      | mask_names = get_param(gcb, 'MaskNames');
      | if strcmp(get_param(gcb, 'io_dir'), 'To Processor'),
      |     mask_enables{ismember(mask_names, 'sample_period')} = 'off';
      | else
      |     mask_enables{ismember(mask_names, 'sample_period')} = 'on';
      | end
      | set_param(gcb, 'MaskEnables', mask_enables);
      mask DialogControl ParameterTabVar0 Prompt: Setup
  ss0 : Subsystem
  ss1 : Subsystem
  ss10 : Subsystem
  ss11 : Subsystem
  ss12 : Subsystem
  ss13 : Subsystem
  ss14 : Subsystem
  ss15 : Subsystem
  ss2 : Subsystem
  ss3 : Subsystem
  ss4 : Subsystem
  ss5 : Subsystem
  ss6 : Subsystem
  ss7 : Subsystem
  ss8 : Subsystem
  ss9 : Subsystem
  ss_lsb : Subsystem
  ss_msb : Subsystem
  wires:
  Counter/1 -> Slice/1
  Slice/1 -> ROM/1
  reg_in/1(in_reg) -> Delay/1
  Delay/1 -> reg_out/1(out_reg)
  ROM/1 -> Delay1/1
  Delay1/1 -> gpio/1
  ROM1/1 -> Delay2/1
  Slice1/1 -> ROM1/1
  Counter1/1 -> Slice1/1
  Delay2/1 -> gpio1/1
  Constant/1 -> htg_adc_yb/1(m00_axis_tready)
  Constant1/1 -> htg_adc_yb/2(m01_axis_tready)
  Constant2/1 -> htg_adc_yb/3(m02_axis_tready)
  Constant3/1 -> htg_adc_yb/4(m03_axis_tready)
  Constant4/1 -> htg_adc_yb/5(m10_axis_tready)
  Constant5/1 -> htg_adc_yb/6(m11_axis_tready)
  Constant6/1 -> htg_adc_yb/7(m12_axis_tready)
  Constant7/1 -> htg_adc_yb/8(m13_axis_tready)
  Constant8/1 -> htg_adc_yb/9(m20_axis_tready)
  Constant9/1 -> htg_adc_yb/10(m21_axis_tready)
  Constant10/1 -> htg_adc_yb/11(m22_axis_tready)
  Constant11/1 -> htg_adc_yb/12(m23_axis_tready)
  Constant14/1 -> htg_adc_yb/13(m30_axis_tready)
  Constant15/1 -> htg_adc_yb/14(m31_axis_tready)
  Constant12/1 -> htg_adc_yb/15(m32_axis_tready)
  Constant13/1 -> htg_adc_yb/16(m33_axis_tready)
  Constant17/1 -> deadbeef/1(out_reg)
  count_rst/1(in_reg) -> Counter2/1
  Counter2/1 -> Delay3/1
  Delay3/1 -> count_out/1(out_reg)
  adc_rstn/1(in_reg) -> htg_adc_yb/17(rstn)
  htg_adc_yb/1(m00_axis_tdata) -> munge/1(din)
  htg_adc_yb/2(m00_axis_tvalid) -> ss_msb/2(vld), ss_lsb/2(vld), ss0/2(vld)
  htg_adc_yb/3(m01_axis_tdata) -> munge1/1(din)
  htg_adc_yb/4(m01_axis_tvalid) -> ss1/2(vld)
  htg_adc_yb/5(m02_axis_tdata) -> munge2/1(din)
  htg_adc_yb/6(m02_axis_tvalid) -> ss2/2(vld)
  htg_adc_yb/7(m03_axis_tdata) -> munge3/1(din)
  htg_adc_yb/8(m03_axis_tvalid) -> ss3/2(vld)
  htg_adc_yb/9(m10_axis_tdata) -> munge4/1(din)
  htg_adc_yb/10(m10_axis_tvalid) -> ss4/2(vld)
  htg_adc_yb/11(m11_axis_tdata) -> munge5/1(din)
  htg_adc_yb/12(m11_axis_tvalid) -> ss5/2(vld)
  htg_adc_yb/13(m12_axis_tdata) -> munge6/1(din)
  htg_adc_yb/14(m12_axis_tvalid) -> ss6/2(vld)
  htg_adc_yb/15(m13_axis_tdata) -> munge7/1(din)
  htg_adc_yb/16(m13_axis_tvalid) -> ss7/2(vld)
  htg_adc_yb/17(m20_axis_tdata) -> munge8/1(din)
  htg_adc_yb/18(m20_axis_tvalid) -> ss8/2(vld)
  htg_adc_yb/19(m21_axis_tdata) -> munge9/1(din)
  htg_adc_yb/20(m21_axis_tvalid) -> ss9/2(vld)
  htg_adc_yb/21(m22_axis_tdata) -> munge10/1(din)
  htg_adc_yb/22(m22_axis_tvalid) -> ss10/2(vld)
  htg_adc_yb/23(m23_axis_tdata) -> munge11/1(din)
  htg_adc_yb/24(m23_axis_tvalid) -> ss11/2(vld)
  htg_adc_yb/25(m30_axis_tdata) -> munge12/1(din)
  htg_adc_yb/26(m30_axis_tvalid) -> ss12/2(vld)
  htg_adc_yb/27(m31_axis_tdata) -> munge13/1(din)
  htg_adc_yb/28(m31_axis_tvalid) -> ss13/2(vld)
  htg_adc_yb/29(m32_axis_tdata) -> munge14/1(din)
  htg_adc_yb/30(m32_axis_tvalid) -> ss14/2(vld)
  htg_adc_yb/31(m33_axis_tdata) -> munge15/1(din)
  htg_adc_yb/32(m33_axis_tvalid) -> ss15/2(vld)
  munge/1(dout) -> Slice3/1, Slice2/1, ss0/1(din)
  munge1/1(dout) -> ss1/1(din)
  munge2/1(dout) -> ss2/1(din)
  munge3/1(dout) -> ss3/1(din)
  munge4/1(dout) -> ss4/1(din)
  munge5/1(dout) -> ss5/1(din)
  munge6/1(dout) -> ss6/1(din)
  munge7/1(dout) -> ss7/1(din)
  munge8/1(dout) -> ss8/1(din)
  munge9/1(dout) -> ss9/1(din)
  munge10/1(dout) -> ss10/1(din)
  munge11/1(dout) -> ss11/1(din)
  munge12/1(dout) -> ss12/1(din)
  munge13/1(dout) -> ss13/1(din)
  munge14/1(dout) -> ss14/1(din)
  munge15/1(dout) -> ss15/1(din)
  Slice2/1 -> ss_lsb/1(din)
  Slice3/1 -> ss_msb/1(din)

== system zrf_test/HTG_ZRF16 ==

== system zrf_test/adc_rstn ==
  convert1_1 : DataTypeConversion  OutDataTypeStr=fixdt('ufix1_En0')  LockScale=on
  convert2_1 : DataTypeConversion  OutDataTypeStr=fixdt('ufix1_En0')  ConvertRealWorld=Stored Integer (SI)  LockScale=on
  gain_1 : Gain
  io_delay : xbsIndex_r4/Delay  rst=off  infoeditControl=Selection of Reset will increase slice count due to use of real FFs and instead of SRLs  en=off  latency=0  reg_retiming=on  dbl_ovrd=off  block_type=delay
  sim_1 : Constant  Value=0
  slice_reg : xbsIndex_r4/Slice  nbits=1  boolean_output=on  mode=Lower Bit Location + Width  bit1=0  base1=MSB of Input  bit0=0  base0=LSB of Input  dbl_ovrd=off  block_type=slice
  zrf_test_adc_rstn_user_data_out : xbsIndex_r4/Gateway In  gui_display_data_type=Fixed-point  arith_type=Unsigned  n_bits=32  bin_pt=0  preci_type=Single  exp_width=8  frac_width=24  rows=1  columns=1  quantization="Round  (unbiased: +/- Inf)"  overflow=Saturate  period=1  UseAsADC=off  ADCChannel='1'  interface=None  automatic_assignment=on  address_offset=hex2dec('00')  intf_name=''  intf_description=''  default_value=0  timing_constraint=None  locs_specified=off  LOCs={}  io_standard={}  inherit_from_input=off  hdl_port=on  dbl_ovrd=off  block_type=gatewayin
  in_reg : Outport
  wires:
  zrf_test_adc_rstn_user_data_out/1 -> io_delay/1
  sim_1/1 -> convert1_1/1
  convert1_1/1 -> convert2_1/1
  convert2_1/1 -> gain_1/1
  gain_1/1 -> zrf_test_adc_rstn_user_data_out/1
  io_delay/1 -> slice_reg/1
  slice_reg/1 -> in_reg/1
